simulink model "ddc_specavg"  (R2023b)
settings: Solver=VariableStepAuto  StartTime=0.0  StopTime=5e-4  RelTol=1e-3
values from neighbouring files (symbols this model uses):
  Fs = 60e6    (= 60000000)    [ddc_specavg_matlabcode.m]
  hf = fi(h, 1, 12, 11)    [ddc_specavg_matlabcode.m]
undefined symbols (not defined in the file or in its folder): Add, Shift
libraries: dspsrcs4 x1, dsphdlmathfun2 x1, dsphdlxfrm2 x1, dsphdlsigops2 x1
settings Model: Creator=nishi  LastModifiedBy=nishi

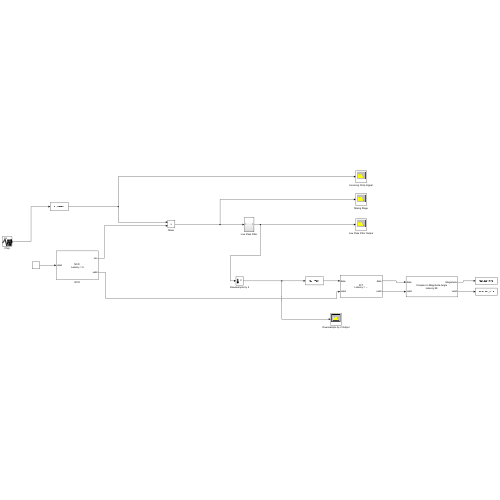
[thumbnail: Simulink's stored preview of the top-level diagram]
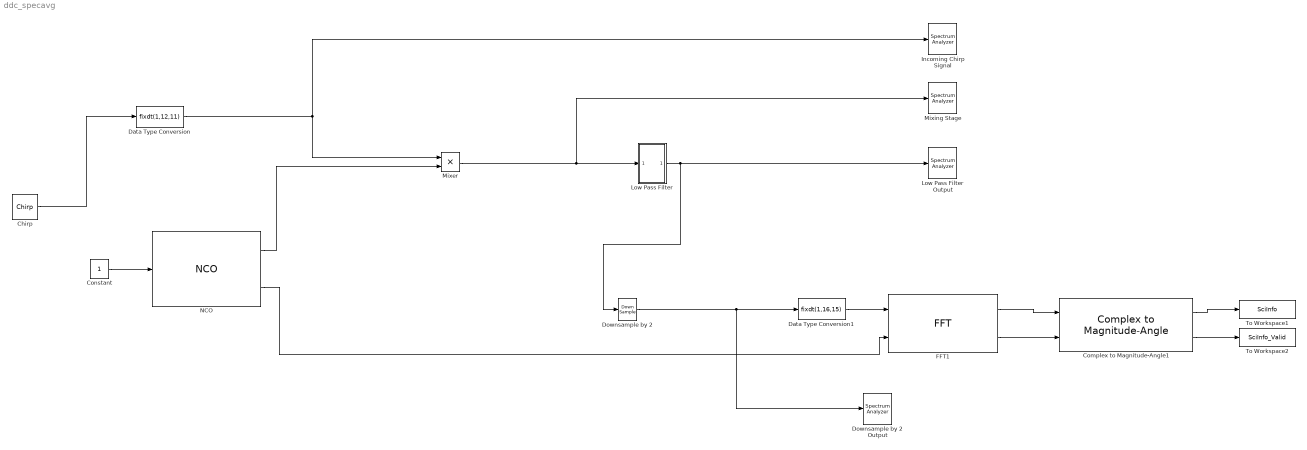
== system ddc_specavg ==
  Chirp : dspsrcs4/Chirp  sweep=Linear  mode=Unidirectional  f0=10e6  f1=20e6  t1=0.00001998  Tsweep=0.00001998  phase=0  Ts=1/Fs  spf=1  datatype=Double  OutputFrames=off
  Complex to Magnitude-Angle1 : dsphdlmathfun2/Complex to Magnitude-Angle  NumIterationsSource=Auto  NumIterations=10  OutputFormat=Magnitude  AngleFormat=Normalized  ScaleOutput=on  ScalingMethod=Shift-Add  SimulateUsing=Code generation
  Constant : Constant  OutDataTypeStr=boolean
  Data Type Conversion : DataTypeConversion  OutDataTypeStr=fixdt(1,12,11)  RndMeth=Floor
  Data Type Conversion1 : DataTypeConversion  OutDataTypeStr=fixdt(1,16,15)  SaturateOnIntegerOverflow=off  RndMeth=Floor
  Downsample by 2 : DownSample  RateOptions=Allow multirate processing
  Downsample by 2 Output : SpectrumAnalyzer  WindowPosition=[389.000000,53.000000,556.000000,366.000000,]  Visible=on  ScopeFrameLocation=window  YLimits=[-54.44708113,2.41421505]
  FFT1 : dsphdlxfrm2/FFT  FFTLength=FFT  Architecture=Streaming Radix 2^2  ComplexMultiplication=Use 4 multipliers and 2 adders  BitReversedOutput=off  BitReversedInput=off  Normalize=off  SimulateUsing=Code generation  RoundingMethod=Floor  ResetInputPort=off  StartOutputPort=off  EndOutputPort=off
  Incoming Chirp Signal : SpectrumAnalyzer  WindowPosition=[365.000000,457.000000,581.000000,366.000000,]  Visible=on  ScopeFrameLocation=window  YLimits=[-42.80600606,8.05668186]
  Low Pass Filter : Subsystem
  Low Pass Filter Output : SpectrumAnalyzer  WindowPosition=[983.000000,57.000000,512.000000,370.000000,]  Visible=on  ScopeFrameLocation=window  YLimits=[-117.8045694,13.08403837]
  Mixer : Product
  Mixing Stage : SpectrumAnalyzer  WindowPosition=[973.000000,472.000000,545.000000,353.000000,]  Visible=on  ScopeFrameLocation=window  YLimits=[-45.45285408,5.04921771]
  NCO : dsphdlsigops2/NCO  PhaseIncrementSource=Property  PhaseIncrement=phIncr  PhaseOffsetSource=Property  PhaseOffset=phOff  DitherSource=Property  NumDitherBits=ditherBits  SamplesPerFrame=1  LUTCompress=off  ResetAction=off  Waveform=Cosine  PhasePort=off  SimulateUsing=Code generation  AccumulatorWL=N  PhaseQuantization=on  NumQuantizerAccumulatorBits=Q  OutputDataType=Binary point scaling  OutputWL=16  OutputFL=14
      settings: LibrarySourceBlock=dsphdlsrcs2/NCO
  To Workspace1 : ToWorkspace  VariableName=SciInfo  SampleTime=-1
      settings: Save2DSignal=2-D array (concatenate along first dimension)
  To Workspace2 : ToWorkspace  VariableName=SciInfo_Valid  SampleTime=-1
      settings: Save2DSignal=2-D array (concatenate along first dimension)
  wires:
  Data Type Conversion/1 -> Incoming Chirp Signal/1, Mixer/1
  Low Pass Filter/1(Out1) -> Downsample by 2/1, Low Pass Filter Output/1
  Mixer/1 -> Mixing Stage/1, Low Pass Filter/1(In1)
  NCO/1 -> Mixer/2
  Constant/1 -> NCO/1
  NCO/2 -> FFT1/2
  Chirp/1 -> Data Type Conversion/1
  Complex to Magnitude-Angle1/2 -> To Workspace2/1
  Complex to Magnitude-Angle1/1 -> To Workspace1/1
  Downsample by 2/1 -> Data Type Conversion1/1, Downsample by 2 Output/1
  Data Type Conversion1/1 -> FFT1/1
  FFT1/1 -> Complex to Magnitude-Angle1/1
  FFT1/2 -> Complex to Magnitude-Angle1/2

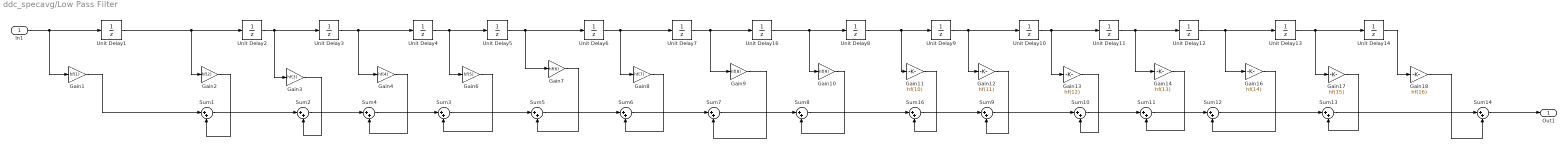
== system ddc_specavg/Low Pass Filter ==
  In1 : Inport
  Gain1 : Gain  Gain=hf(1)
  Gain10 : Gain  Gain=hf(9)
  Gain11 : Gain  Gain=hf(10)
  Gain12 : Gain  Gain=hf(11)
  Gain13 : Gain  Gain=hf(12)
  Gain14 : Gain  Gain=hf(13)
  Gain16 : Gain  Gain=hf(14)
  Gain17 : Gain  Gain=hf(15)
  Gain18 : Gain  Gain=hf(16)
  Gain2 : Gain  Gain=hf(2)
  Gain3 : Gain  Gain=hf(3)
  Gain4 : Gain  Gain=hf(4)
  Gain6 : Gain  Gain=hf(5)
  Gain7 : Gain  Gain=hf(6)
  Gain8 : Gain  Gain=hf(7)
  Gain9 : Gain  Gain=hf(8)
  Sum{1..14,16} (15 alike) : Sum  Inputs=|++
  Unit Delay{1..14,16} (15 alike) : UnitDelay  SampleTime=-1  HasFrameUpgradeWarning=on
  Out1 : Outport
  wires:
  Sum2/1 -> Sum4/1
  Sum7/1 -> Sum8/1
  Gain6/1 -> Sum3/2
  Unit Delay3/1 -> Unit Delay4/1, Gain4/1
  Unit Delay5/1 -> Unit Delay6/1, Gain7/1
  Unit Delay8/1 -> Unit Delay9/1, Gain11/1
  Sum16/1 -> Sum9/1
  Gain14/1 -> Sum11/2
  Unit Delay16/1 -> Unit Delay8/1, Gain10/1
  Unit Delay9/1 -> Unit Delay10/1, Gain12/1
  Unit Delay6/1 -> Unit Delay7/1, Gain8/1
  In1/1 -> Unit Delay1/1, Gain1/1
  Gain8/1 -> Sum6/2
  Sum6/1 -> Sum7/1
  Sum13/1 -> Sum14/1
  Unit Delay2/1 -> Unit Delay3/1, Gain3/1
  Unit Delay11/1 -> Unit Delay12/1, Gain14/1
  Unit Delay4/1 -> Unit Delay5/1, Gain6/1
  Sum12/1 -> Sum13/1
  Gain18/1 -> Sum14/2
  Unit Delay7/1 -> Unit Delay16/1, Gain9/1
  Unit Delay14/1 -> Gain18/1
  Gain11/1 -> Sum16/2
  Sum3/1 -> Sum5/1
  Sum14/1 -> Out1/1
  Sum10/1 -> Sum11/1
  Unit Delay10/1 -> Unit Delay11/1, Gain13/1
  Unit Delay1/1 -> Gain2/1, Unit Delay2/1
  Sum4/1 -> Sum3/1
  Gain3/1 -> Sum2/2
  Gain13/1 -> Sum10/2
  Gain1/1 -> Sum1/1
  Gain10/1 -> Sum8/2
  Gain9/1 -> Sum7/2
  Gain16/1 -> Sum12/2
  Gain12/1 -> Sum9/2
  Gain7/1 -> Sum5/2
  Gain17/1 -> Sum13/2
  Sum8/1 -> Sum16/1
  Unit Delay12/1 -> Unit Delay13/1, Gain16/1
  Gain4/1 -> Sum4/2
  Sum11/1 -> Sum12/1
  Unit Delay13/1 -> Unit Delay14/1, Gain17/1
  Gain2/1 -> Sum1/2
  Sum9/1 -> Sum10/1
  Sum1/1 -> Sum2/1
  Sum5/1 -> Sum6/1
